simulink model "ADDPLANT_Harness1"  (R2024b)
settings: Solver=VariableStepAuto  StartTime=0.0  StopTime=10.0  RelTol=1e-3
settings Model: Creator=User  LastModifiedBy=User

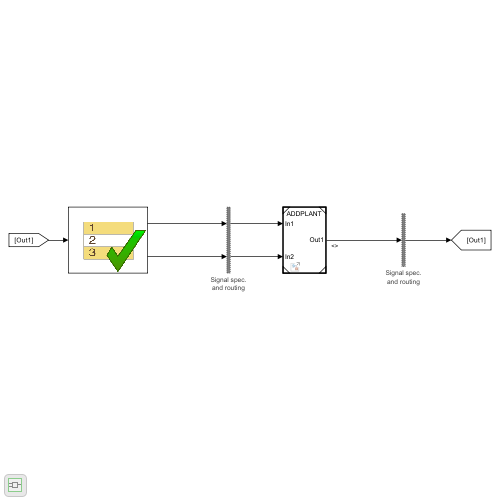
[thumbnail: Simulink's stored preview of the top-level diagram]
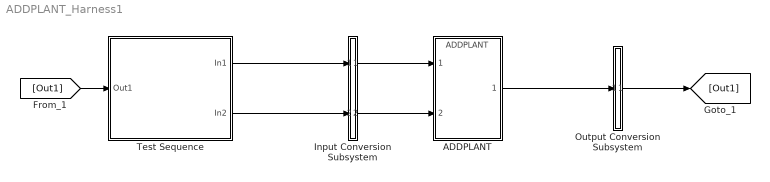
== system ADDPLANT_Harness1 ==
  ADDPLANT : ModelReference  ModelNameDialog=ADDPLANT  SimulationMode=Normal  ModelReferenceVersion=1.1
  Input Conversion Subsystem : Subsystem  Tag=__SLT_ICS__  Description=|
      | Signal spec.
      | and routing
      settings: AttributesFormatString=%<Description>
  Output Conversion Subsystem : Subsystem  Tag=__SLT_OCS__  Description=|
      | Signal spec.
      | and routing
      settings: AttributesFormatString=%<Description>
  Test Sequence : Test Sequence  TreatAsAtomicUnit=on
  wires:
  Test Sequence/1(In1) -> Input Conversion Subsystem/1(Inport_1)
  Test Sequence/2(In2) -> Input Conversion Subsystem/2(Inport_2)
  [Out1] -> Test Sequence/1(Out1)
  Output Conversion Subsystem/1(Outport_1) -> [Out1]
  Input Conversion Subsystem/1(Outport_1) -> ADDPLANT/1
  Input Conversion Subsystem/2(Outport_2) -> ADDPLANT/2
  ADDPLANT/1 -> Output Conversion Subsystem/1(Inport_1)

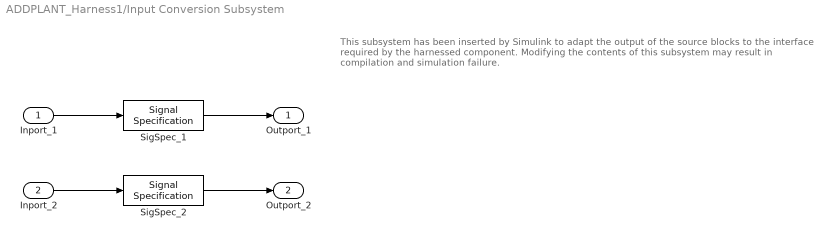
== system ADDPLANT_Harness1/Input Conversion Subsystem ==
  note: This subsystem has been inserted by Simulink to adapt the output of the source blocks to the interface required by the harnessed component.
      |  Modifying the contents of this subsystem may result in compilation and simulation failure.
  Inport_1 : Inport
  Inport_2 : Inport  Port=2
  SigSpec_1 : SignalSpecification  OutDataTypeStr=double  Dimensions=[1]  SampleTime=[-1, 0]
  SigSpec_2 : SignalSpecification  OutDataTypeStr=double  Dimensions=[1]  SampleTime=[-1, 0]
  Outport_1 : Outport
  Outport_2 : Outport  Port=2
  wires:
  SigSpec_1/1 -> Outport_1/1
  Inport_1/1 -> SigSpec_1/1
  SigSpec_2/1 -> Outport_2/1
  Inport_2/1 -> SigSpec_2/1

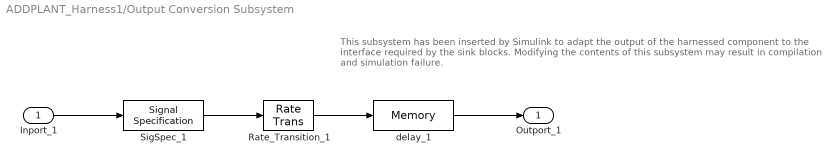
== system ADDPLANT_Harness1/Output Conversion Subsystem ==
  note: This subsystem has been inserted by Simulink to adapt the output of the harnessed component to the interface required by the sink blocks.
      |  Modifying the contents of this subsystem may result in compilation and simulation failure.
  Inport_1 : Inport
  Rate_Transition_1 : RateTransition  OutPortSampleTimeOpt=Inherit
  SigSpec_1 : SignalSpecification  OutDataTypeStr=double  Dimensions=[1]
  delay_1 : Memory
  Outport_1 : Outport
  wires:
  Inport_1/1 -> SigSpec_1/1
  SigSpec_1/1 -> Rate_Transition_1/1
  Rate_Transition_1/1 -> delay_1/1
  delay_1/1 -> Outport_1/1

== stateflow chart ADDPLANT_Harness1/Test Sequence ==
  state Scenario_1
    state Run
      %% Initialize data outputs.
      In1 = 1;
      In2 = 2;
    (default) -> Run
  (default) -> Scenario_1 : {assert(Active_Scenario_Index == 1,'The value of Scenario Parameter ''Active_Scenario_Index'' is not valid. Use the index of the scenario to specify it.')}
  data: Out1 input double size=[1]; In1 output double size=[1]; In2 output double size=[1]; Active_Scenario_Index parameter =1
